simulink model "parnas_pacemaker_v7"  (R2017b)
settings: Solver=FixedStepAuto  StartTime=0.0  StopTime=10  FixedStep=1E-3  RelTol=1e-3  EnableMultiTasking=on
undefined symbols (not defined in the file): A0, A1, D0, D1, D10, D11, D12, D13, D2, D3, D4, D5, D6, D7, D8, D9, magnitude, PTA0, PTA1, PTA2, PTB2, PTB23, PTB3, PTB9, PTC16, PTC17, PTC2, PTC3, PTC4, PTD0, PTD1, PTD2, PTD3
libraries: frdmk64flib x19, etargetslib x2
settings Model: ExtModeTrigDuration=5  Creator=fahadbandali  LastModifiedBy=fahadbandali
settings OptimizationCC: PassReuseOutputArgsAs=Individual arguments  MaxStackSize=64
settings DebuggingCC: ParameterTunabilityLossMsg=error
settings HardwareCC: ProdBitPerPointer=32  ProdBitPerSizeT=32  ProdBitPerPtrDiffT=32  ProdLargestAtomicInteger=Long  ProdLargestAtomicFloat=Double  ProdWordSize=32  ProdHWDeviceType=ARM Compatible->ARM Cortex
settings SFSimCC: MATLABDynamicMemAlloc=off
settings RTWCC: SystemTargetFile=ert.tlc  HardwareBoard=NXP FRDM-K64F  TemplateMakefile=ert_default_tmf  GenerateReport=on  Toolchain=GNU Tools for ARM Embedded Processors  IncludeHyperlinkInReport=on  LaunchReport=on  GenerateTraceInfo=on  GenerateTraceReport=on  GenerateTraceReportSl=on  GenerateTraceReportSf=on  GenerateTraceReportEml=on
settings CodeAppCC: ForceParamTrailComments=on  IgnoreCustomStorageClasses=off  OperatorAnnotations=on  SimulinkDataObjDesc=on  SFDataObjDesc=on  InsertBlockDesc=on

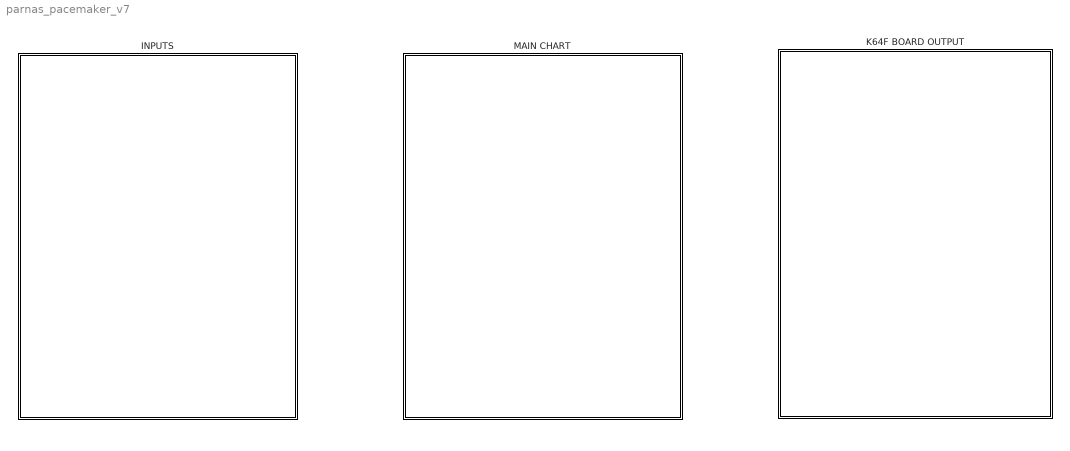
== system parnas_pacemaker_v7 ==
  "INPUTS " : Subsystem
  "K64F BOARD OUTPUT " : Subsystem
  "MAIN CHART " : Subsystem

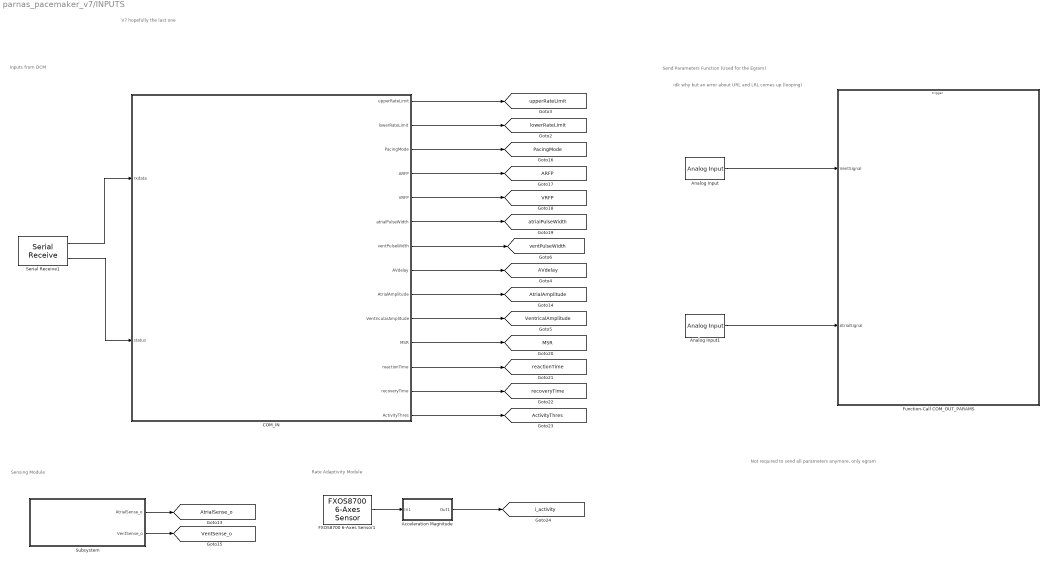
== system parnas_pacemaker_v7/INPUTS  ==
  note: Not required to send all parameters anymore, only egram
  note: V7 hopefully the last one
  note: idk why but an error about URL and LRL comes up (looping)
  note: Send Parameters Function (Used for the Egram)
  note: Inputs from DCM
  note: Rate Adaptivity Module
  note: Sensing Module
  Acceleration Magnitude : Subsystem
  Analog Input : frdmk64flib/Analog Input  Whichpin=PTB3 (A1)  SampleTime=-1
      settings: SourceProductName=Simulink Coder Support Package for NXP FRDM-K64F Board
  Analog Input1 : frdmk64flib/Analog Input  Whichpin=PTB2 (A0)  SampleTime=-1
      settings: SourceProductName=Simulink Coder Support Package for NXP FRDM-K64F Board
  COM_IN : Stateflow chart  TreatAsAtomicUnit=on
  FXOS8700 6-Axes Sensor1 : frdmk64flib/FXOS8700 6-Axes Sensor  Activesensor=Accelerometer only  ODR=800Hz  HybridODR=400Hz  Accelfullrange=-4g to +4g  SampleTime=-1
      settings: SourceProductName=Simulink Coder Support Package for NXP FRDM-K64F Board
  Function-Call COM_OUT_PARAMS : Subsystem  TreatAsAtomicUnit=on
  Serial Receive1 : frdmk64flib/Serial Receive  SCIModule=0  Baudrate=uint32(9600)  Parity=None  StopBits=1  HardwareFlowControl=None  ByteOrder=LittleEndian  DataType=uint8  DataLength=30  BlockingMode=off  OutputStatus=on  SampleTime=-1
      settings: SourceProductName=Simulink Coder Support Package for NXP FRDM-K64F Board
  Subsystem : Subsystem
  tag scope: ARFP=global, AVdelay=global, ActivityThres=global, AtrialAmplitude=global, AtrialSense_o=global, MSR=global, PacingMode=global, VRFP=global, VentSense_o=global, VentricalAmplitude=global, atrialPulseWidth=global, i_activity=global, lowerRateLimit=global, reactionTime=global, recoveryTime=global, upperRateLimit=global, ventPulseWidth=global
  wires:
  Subsystem/2("VentSense_o ") -> [VentSense_o]
  Subsystem/1("AtrialSense_o ") -> [AtrialSense_o]
  FXOS8700 6-Axes Sensor1/1 -> Acceleration Magnitude/1(In1)
  COM_IN/3(PacingMode) -> [PacingMode]
  COM_IN/4(ARFP) -> [ARFP]
  COM_IN/5(VRFP) -> [VRFP]
  COM_IN/6(atrialPulseWidth) -> [atrialPulseWidth]
  COM_IN/8(AVdelay) -> [AVdelay]
  COM_IN/9(AtrialAmplitude) -> [AtrialAmplitude]
  COM_IN/10(VentricularAmplitude) -> [VentricalAmplitude]
  COM_IN/11(MSR) -> [MSR]
  COM_IN/12(reactionTime) -> [reactionTime]
  COM_IN/13(recoveryTime) -> [recoveryTime]
  COM_IN/14(ActivityThres) -> [ActivityThres]
  Serial Receive1/1 -> COM_IN/1(rxdata)
  Serial Receive1/2 -> COM_IN/2(status)
  Analog Input1/1 -> Function-Call COM_OUT_PARAMS/2(AtrialSignal)
  Analog Input/1 -> Function-Call COM_OUT_PARAMS/1(VentSignal)
  COM_IN/1(upperRateLimit) -> [upperRateLimit]
  COM_IN/2(lowerRateLimit) -> [lowerRateLimit]
  COM_IN/7(ventPulseWidth) -> [ventPulseWidth]
  Acceleration Magnitude/1(Out1) -> [i_activity]

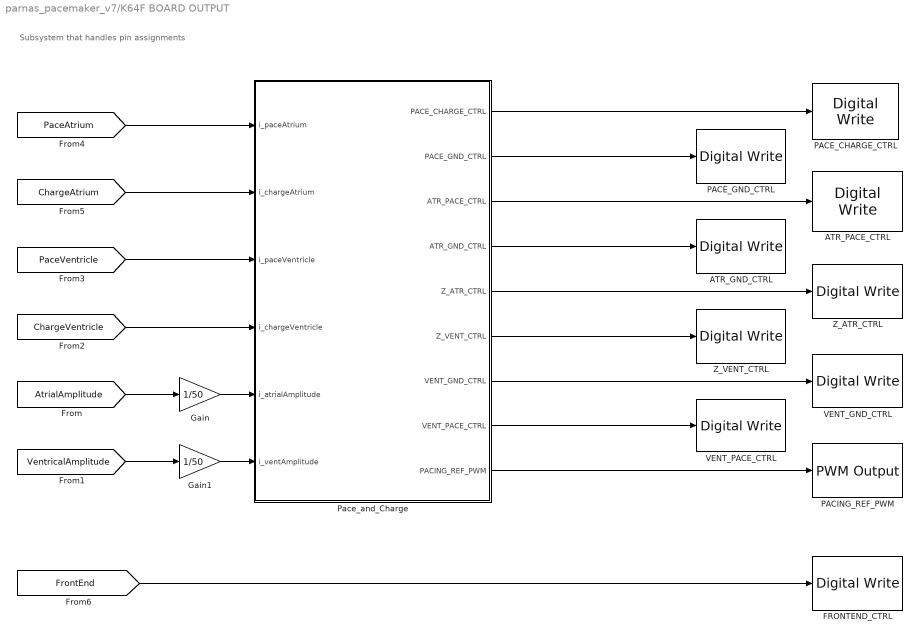
== system parnas_pacemaker_v7/K64F BOARD OUTPUT  ==
  note: Subsystem that handles pin assignments
  " ATR_GND_CTRL" : frdmk64flib/Digital Write  Whichpin=PTD2 (D11)
      settings: SourceProductName=Simulink Coder Support Package for NXP FRDM-K64F Board
  " ATR_PACE_CTRL" : frdmk64flib/Digital Write  Whichpin=PTA0 (D8)
      settings: SourceProductName=Simulink Coder Support Package for NXP FRDM-K64F Board
  " PACE_GND_CTRL" : frdmk64flib/Digital Write  Whichpin=PTD0 (D10)
      settings: SourceProductName=Simulink Coder Support Package for NXP FRDM-K64F Board
  " VENT_PACE_CTRL" : frdmk64flib/Digital Write  Whichpin=PTC4 (D9)
      settings: SourceProductName=Simulink Coder Support Package for NXP FRDM-K64F Board
  "FRONTEND_CTRL " : frdmk64flib/Digital Write  Whichpin=PTD1 (D13)
      settings: SourceProductName=Simulink Coder Support Package for NXP FRDM-K64F Board
  Gain : Gain  Gain=1/50  OutDataTypeStr=uint16
  Gain1 : Gain  Gain=1/50  OutDataTypeStr=uint16
  PACE_CHARGE_CTRL : frdmk64flib/Digital Write  Whichpin=PTB9 (D2)
      settings: SourceProductName=Simulink Coder Support Package for NXP FRDM-K64F Board
  PACING_REF_PWM : frdmk64flib/PWM Output  Whichpin=PTA2 (D5)  InitialFrequency=2000  InitialDutyCycle=0
      settings: SourceProductName=Simulink Coder Support Package for NXP FRDM-K64F Board
  Pace_and_Charge : Stateflow chart  TreatAsAtomicUnit=on
  "VENT_GND_CTRL " : frdmk64flib/Digital Write  Whichpin=PTD3 (D12)
      settings: SourceProductName=Simulink Coder Support Package for NXP FRDM-K64F Board
  Z_ATR_CTRL : frdmk64flib/Digital Write  Whichpin=PTB23 (D4)
      settings: SourceProductName=Simulink Coder Support Package for NXP FRDM-K64F Board
  Z_VENT_CTRL : frdmk64flib/Digital Write  Whichpin=PTC3 (D7)
      settings: SourceProductName=Simulink Coder Support Package for NXP FRDM-K64F Board
  wires:
  Pace_and_Charge/1(PACE_CHARGE_CTRL) -> PACE_CHARGE_CTRL/1
  Pace_and_Charge/2(PACE_GND_CTRL) -> " PACE_GND_CTRL"/1
  Pace_and_Charge/3(ATR_PACE_CTRL) -> " ATR_PACE_CTRL"/1
  [PaceAtrium] -> Pace_and_Charge/1(i_paceAtrium)
  [PaceVentricle] -> Pace_and_Charge/3(i_paceVentricle)
  Pace_and_Charge/4(ATR_GND_CTRL) -> " ATR_GND_CTRL"/1
  Pace_and_Charge/5(Z_ATR_CTRL) -> Z_ATR_CTRL/1
  Pace_and_Charge/6(Z_VENT_CTRL) -> Z_VENT_CTRL/1
  Pace_and_Charge/7(VENT_GND_CTRL) -> "VENT_GND_CTRL "/1
  Pace_and_Charge/8(VENT_PACE_CTRL) -> " VENT_PACE_CTRL"/1
  Pace_and_Charge/9(PACING_REF_PWM) -> PACING_REF_PWM/1
  [ChargeAtrium] -> Pace_and_Charge/2(i_chargeAtrium)
  [ChargeVentricle] -> Pace_and_Charge/4(i_chargeVentricle)
  [AtrialAmplitude] -> Gain/1
  Gain/1 -> Pace_and_Charge/5(i_atrialAmplitude)
  [VentricalAmplitude] -> Gain1/1
  Gain1/1 -> Pace_and_Charge/6(i_ventAmplitude)
  [FrontEnd] -> "FRONTEND_CTRL "/1

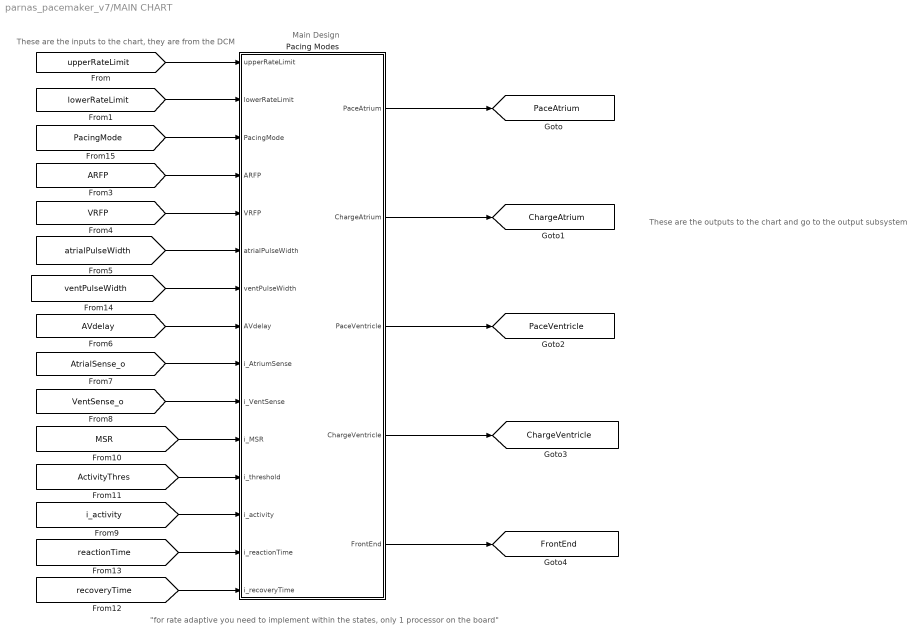
== system parnas_pacemaker_v7/MAIN CHART  ==
  note: These are the outputs to the chart and go to the output subsystem
  note: These are the inputs to the chart, they are from the DCM
  note: Main Design
  note: "for rate adaptive you need to implement within the states, only 1 processor on the board"
  Pacing Modes : Stateflow chart  TreatAsAtomicUnit=on
  tag scope: ChargeAtrium=global, ChargeVentricle=global, FrontEnd=global, PaceAtrium=global, PaceVentricle=global
  wires:
  [PacingMode] -> Pacing Modes/3(PacingMode)
  [AVdelay] -> Pacing Modes/8(AVdelay)
  [VentSense_o] -> Pacing Modes/10(i_VentSense)
  [upperRateLimit] -> Pacing Modes/1(upperRateLimit)
  Pacing Modes/3(PaceVentricle) -> [PaceVentricle]
  [atrialPulseWidth] -> Pacing Modes/6(atrialPulseWidth)
  Pacing Modes/5(FrontEnd) -> [FrontEnd]
  [AtrialSense_o] -> Pacing Modes/9(i_AtriumSense)
  [VRFP] -> Pacing Modes/5(VRFP)
  [ARFP] -> Pacing Modes/4(ARFP)
  Pacing Modes/2(ChargeAtrium) -> [ChargeAtrium]
  Pacing Modes/1(PaceAtrium) -> [PaceAtrium]
  [MSR] -> Pacing Modes/11(i_MSR)
  [ActivityThres] -> Pacing Modes/12(i_threshold)
  [lowerRateLimit] -> Pacing Modes/2(lowerRateLimit)
  [i_activity] -> Pacing Modes/13(i_activity)
  Pacing Modes/4(ChargeVentricle) -> [ChargeVentricle]
  [ventPulseWidth] -> Pacing Modes/7(ventPulseWidth)
  [recoveryTime] -> Pacing Modes/15(i_recoveryTime)
  [reactionTime] -> Pacing Modes/14(i_reactionTime)

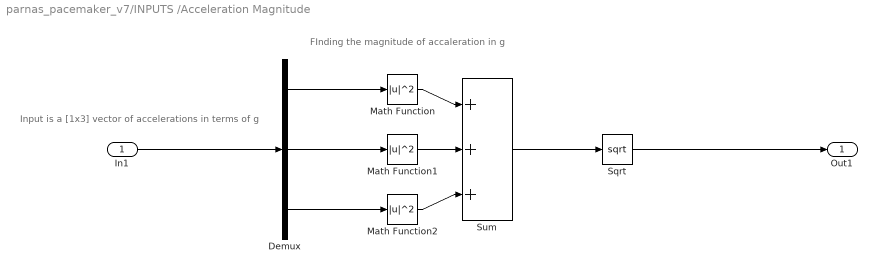
== system parnas_pacemaker_v7/INPUTS /Acceleration Magnitude ==
  note: FInding the magnitude of accaleration in g
  note: Input is a [1x3] vector of accelerations in terms of g
  In1 : Inport
  Demux : Demux  Outputs=3
  Math Function : Math  Operator=magnitude^2  OutDataTypeStr=double  SaturateOnIntegerOverflow=on
  Math Function1 : Math  Operator=magnitude^2  OutDataTypeStr=double  SaturateOnIntegerOverflow=on
  Math Function2 : Math  Operator=magnitude^2  OutDataTypeStr=double  SaturateOnIntegerOverflow=on
  Sqrt : Sqrt  OutputSignalType=real  OutDataTypeStr=uint16  SaturateOnIntegerOverflow=on
  Sum : Sum  Inputs=+|+|+  OutDataTypeStr=double
  Out1 : Outport  OutDataTypeStr=uint16
  wires:
  In1/1 -> Demux/1
  Demux/1 -> Math Function/1
  Demux/3 -> Math Function2/1
  Demux/2 -> Math Function1/1
  Math Function/1 -> Sum/1
  Math Function1/1 -> Sum/2
  Math Function2/1 -> Sum/3
  Sum/1 -> Sqrt/1
  Sqrt/1 -> Out1/1

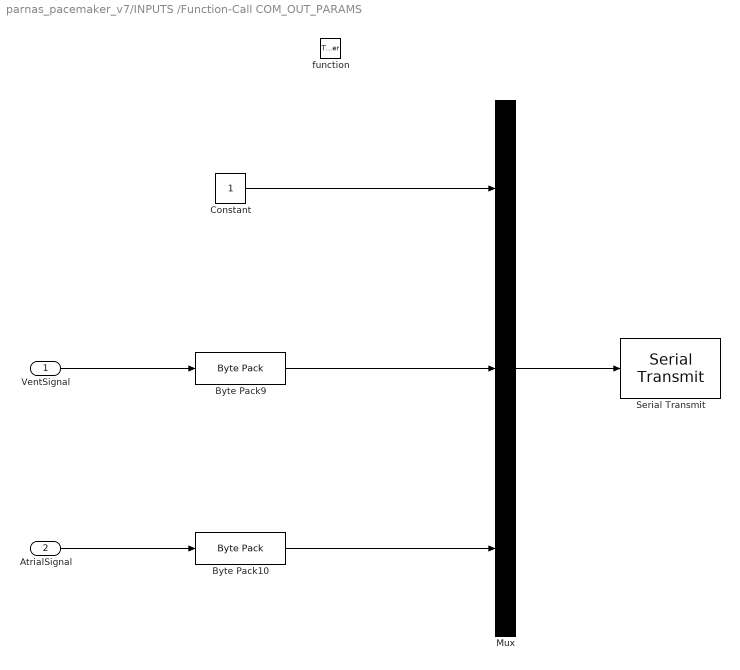
== system parnas_pacemaker_v7/INPUTS /Function-Call COM_OUT_PARAMS ==
  VentSignal : Inport
  AtrialSignal : Inport  Port=2
  function : TriggerPort  TriggerType=function-call  IsSimulinkFunction=on  FunctionName=eegram  VariantControl=Variant
  Byte Pack10 : etargetslib/Byte Pack  datatypes={'double'}  byteAlign=1
  Byte Pack9 : etargetslib/Byte Pack  datatypes={'double'}  byteAlign=1
  Constant : Constant  OutDataTypeStr=uint8
  Mux : Mux  Inputs=3
  Serial Transmit : frdmk64flib/Serial Transmit  SCIModule=0  Baudrate=uint32(9600)  Parity=None  StopBits=1  HardwareFlowControl=None  ByteOrder=LittleEndian  BlockingMode=on  OutputStatus=off
      settings: SourceProductName=Simulink Coder Support Package for NXP FRDM-K64F Board
  wires:
  Mux/1 -> Serial Transmit/1
  Byte Pack9/1 -> Mux/2
  AtrialSignal/1 -> Byte Pack10/1
  VentSignal/1 -> Byte Pack9/1
  Byte Pack10/1 -> Mux/3
  Constant/1 -> Mux/1

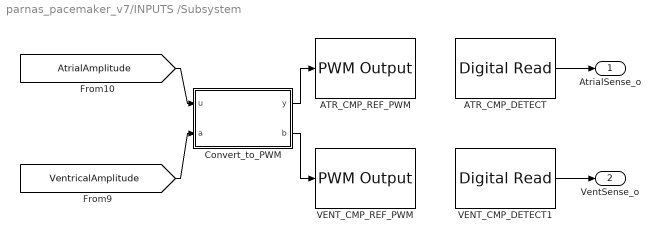
== system parnas_pacemaker_v7/INPUTS /Subsystem ==
  " ATR_CMP_DETECT" : frdmk64flib/Digital Read  Whichpin=PTC16 (D0)  SampleTime=-1
      settings: SourceProductName=Simulink Coder Support Package for NXP FRDM-K64F Board
  " VENT_CMP_DETECT1" : frdmk64flib/Digital Read  Whichpin=PTC17 (D1)  SampleTime=-1
      settings: SourceProductName=Simulink Coder Support Package for NXP FRDM-K64F Board
  ATR_CMP_REF_PWM : frdmk64flib/PWM Output  Whichpin=PTC2 (D6)  InitialFrequency=2000  InitialDutyCycle=0
      settings: SourceProductName=Simulink Coder Support Package for NXP FRDM-K64F Board
  Convert_to_PWM : MATLAB Function  TreatAsAtomicUnit=on
  VENT_CMP_REF_PWM : frdmk64flib/PWM Output  Whichpin=PTA1 (D3)  InitialFrequency=2000  InitialDutyCycle=0
      settings: SourceProductName=Simulink Coder Support Package for NXP FRDM-K64F Board
  "AtrialSense_o " : Outport  OutDataTypeStr=boolean
  "VentSense_o " : Outport  Port=2  OutDataTypeStr=boolean
  wires:
  " ATR_CMP_DETECT"/1 -> "AtrialSense_o "/1
  [VentricalAmplitude] -> Convert_to_PWM/2(a)
  Convert_to_PWM/1(y) -> ATR_CMP_REF_PWM/1
  " VENT_CMP_DETECT1"/1 -> "VentSense_o "/1
  [AtrialAmplitude] -> Convert_to_PWM/1(u)
  Convert_to_PWM/2(b) -> VENT_CMP_REF_PWM/1

== stateflow chart parnas_pacemaker_v7/INPUTS /COM_IN ==
  settings: executeAtInitialization=1
  state SET_PARAM
    entry:
    %setting the values of the parameters
    %using serial communication
    upperRateLimit = typecast(rxdata(3:4), 'uint16');
    lowerRateLimit = typecast(rxdata(5:6), 'uint16');
    PacingMode = typecast(rxdata(7:8), 'uint16');
    ARFP = typecast(rxdata(9:10), 'uint16');
    VRFP = typecast(rxdata(11:12), 'uint16');
    atrialPulseWidth = typecast(rxdata(13:14), 'uint16');
    ventPulseWidth = typecast(rxdata(15:16), 'uint16');
    AVdelay = typecast(rxdata(17:18), 'uint16');
    AtrialAmplitude = typecast(rxdata(19:20), 'uint16');
    VentricularAmplitude = typecast(rxdata(21:22), 'uint16');
    MSR = typecast(rxdata(23:24), 'uint16');
    reactionTime = typecast(rxdata(25:26), 'uint16');
    recoveryTime = typecast(rxdata(27:28), 'uint16');
    ActivityThres = typecast(rxdata(29:30), 'uint16');
    %need to add more parameters
  state INITIAL
    entry:
    %initialize the starting value of the model
    upperRateLimit = 0;
    lowerRateLimit = 0;
    PacingMode = 0;
    ARFP = 0;
    VRFP = 0;
    atrialPulseWidth = 0;
    ventPulseWidth = 0;
    AVdelay = 0;
    AtrialAmplitude = 0;
    VentricularAmplitude = 0;
    MSR = 0;
    reactionTime = 0;
    recoveryTime = 0;
    ActivityThres = 0;
  state STANDBY
    entry:
    %waiting for COM
  state ECHO_PARAM
    entry:
    eegram();
  SET_PARAM -> STANDBY
  (default) -> INITIAL
  (junction 16) -> STANDBY [order 2]
  (junction 17) -> SET_PARAM : [rxdata(2) == hex2dec('55')]
  INITIAL -> STANDBY
  STANDBY -> (junction 16) [order 1] : [status == 0]
  (junction 16) -> (junction 17) [order 1] : [rxdata(1) == hex2dec('16')]
  ECHO_PARAM -> (junction 16) [order 2] : [status == 0]
  ECHO_PARAM -> STANDBY [order 1] : [status == 32]
  STANDBY -> ECHO_PARAM [order 2] : [status == 32]
  data: upperRateLimit output uint16; lowerRateLimit output uint16; PacingMode output uint16; ARFP output uint16; VRFP output uint16; atrialPulseWidth output uint16; ventPulseWidth output uint16; AVdelay output uint16; AtrialAmplitude output uint16; VentricularAmplitude output uint16; rxdata input uint8 size=[30;1]; status input uint8 size=[1;1]; MSR output uint16; reactionTime output uint16; recoveryTime output uint16; ActivityThres output uint16

== stateflow chart parnas_pacemaker_v7/MAIN CHART /Pacing Modes ==
  state DOOR
    note: RATE ADAPTIVE
    state DOO_APACE
      entry:
      PaceAtrium = true;
      PaceVentricle = false;
      ChargeAtrium = false;
      ChargeVentricle = false;
    state DOO_ACHARGE
      entry:
      PaceAtrium = false;
      PaceVentricle = false;
      ChargeAtrium = true;
      ChargeVentricle = false;
      state Start
        entry:
        prevLRL = lowerRateLimitR;
      state FInd_Next_LRL
        entry:
        %finding the response factor (1-16)
        respFactor = i_activity*(4/sqrt(3));
        %finding the new required LRL
        nextLRL = (i_MSR - lowerRateLimit)*(respFactor/16) + lowerRateLimit;
      state Lower_Rate
        entry:
        rateChange = (i_MSR+prevLRL)/2  - lowerRateLimit + 1;
        lowerRateLimitR = floor(prevLRL - (rateChange*60)/(lowerRateLimit*i_recoveryTime));
      state Increase_Rate
        entry:
        rateChange = nextLRL - lowerRateLimit; %find the change in rate
        lowerRateLimitR = prevLRL + (rateChange*60)/(lowerRateLimit*i_reactionTime);
      state Maintain_Rate
        entry:
        lowerRateLimitR  = prevLRL;
      (default) -> DOOR.DOO_ACHARGE.Start
      DOOR.DOO_ACHARGE.Start -> DOOR.DOO_ACHARGE.FInd_Next_LRL [order 1] : [i_activity >= i_threshold]
      DOOR.DOO_ACHARGE.Start -> (junction 443) [order 2] : [i_activity < i_threshold]
      (junction 443) -> DOOR.DOO_ACHARGE.Lower_Rate [order 1] : [prevLRL > lowerRateLimit]
      DOOR.DOO_ACHARGE.FInd_Next_LRL -> DOOR.DOO_ACHARGE.Maintain_Rate [order 2] : [nextLRL <= prevLRL]
      (junction 443) -> DOOR.DOO_ACHARGE.Maintain_Rate [order 2] : [prevLRL <= lowerRateLimit]
      DOOR.DOO_ACHARGE.FInd_Next_LRL -> DOOR.DOO_ACHARGE.Increase_Rate [order 1] : [nextLRL > prevLRL]
    note: RATE ADAPTIVE
    note: DOOR
    note: This state is responsible for pacing both the ventricle and atrium
    state DOO_VPACE
      entry:
      PaceAtrium = false;
      PaceVentricle = true;
      ChargeAtrium = false;
      ChargeVentricle = false;
    state DOO_VCHARGE
      entry:
      PaceAtrium = false;
      PaceVentricle = false;
      ChargeAtrium = false;
      ChargeVentricle = true;
    note: the whole state should be (lowerRateLimit)
    (default) -> DOOR.DOO_ACHARGE : {lowerRateLimitR = lowerRateLimit}
    DOOR.DOO_ACHARGE -> DOOR.DOO_APACE : [after((60000/lowerRateLimitR -AVdelay-ventPulseWidth-atrialPulseWidth), msec)]
    DOOR.DOO_VPACE -> DOOR.DOO_ACHARGE : [after(ventPulseWidth,msec)]
    DOOR.DOO_APACE -> DOOR.DOO_VCHARGE : [after(atrialPulseWidth, msec)]
    DOOR.DOO_VCHARGE -> DOOR.DOO_VPACE : [after(AVdelay,msec)]
  state AAIR
    state AAI_Charge
      entry:
      PaceAtrium = false;
      PaceVentricle = false;
      ChargeVentricle = false;
      ChargeAtrium = true;
      FrontEnd = true;
      state Start
        entry:
        prevLRL = lowerRateLimitR;
      state FInd_Next_LRL
        entry:
        %finding the response factor (1-16)
        respFactor = i_activity*(4/sqrt(3));
        %finding the new required LRL
        nextLRL = (i_MSR - lowerRateLimit)*(respFactor/16) + lowerRateLimit;
      state Lower_Rate
        entry:
        rateChange = (i_MSR+prevLRL)/2  - lowerRateLimit + 1;
        lowerRateLimitR = floor(prevLRL - (rateChange*60)/(lowerRateLimit*i_recoveryTime));
      state Increase_Rate
        entry:
        rateChange = nextLRL - lowerRateLimit; %find the change in rate
        lowerRateLimitR = prevLRL + (rateChange*60)/(lowerRateLimit*i_reactionTime);
      state Maintain_Rate
        entry:
        lowerRateLimitR  = prevLRL;
      (default) -> AAIR.AAI_Charge.Start
      AAIR.AAI_Charge.Start -> AAIR.AAI_Charge.FInd_Next_LRL [order 1] : [i_activity >= i_threshold]
      AAIR.AAI_Charge.Start -> (junction 456) [order 2] : [i_activity < i_threshold]
      (junction 456) -> AAIR.AAI_Charge.Lower_Rate [order 1] : [prevLRL > lowerRateLimit]
      AAIR.AAI_Charge.FInd_Next_LRL -> AAIR.AAI_Charge.Maintain_Rate [order 2] : [nextLRL <= prevLRL]
      (junction 456) -> AAIR.AAI_Charge.Maintain_Rate [order 2] : [prevLRL <= lowerRateLimit]
      AAIR.AAI_Charge.FInd_Next_LRL -> AAIR.AAI_Charge.Increase_Rate [order 1] : [nextLRL > prevLRL]
    note: RATE ADAPTIVE
    note: AAIR
    note: This state is responsible for sensing a pulse in the atrium
        | Initially charging and if a pace is sensed, move to refractor state
        |
        | It stays here for RFP msec and goes back to the initial state,
        | this gives time for the next pulse to appear. If the pulse is not detected
        |
        | It goes to AAI_Pace where a pace is sent and goes back to the refractor state
    state Refractor_AAI
      entry:
      PaceAtrium = false;
      PaceVentricle = false;
      ChargeVentricle = false;
      ChargeAtrium = true;
      FrontEnd = false;
    state AAI_Pace
      entry:
      ChargeAtrium = false;
      ChargeVentricle = false;
      PaceVentricle = false;
      PaceAtrium = true;
      FrontEnd = false;
    (default) -> AAIR.AAI_Charge : {lowerRateLimitR = lowerRateLimit}
    AAIR.AAI_Charge -> AAIR.Refractor_AAI [order 2] : [i_AtriumSense == true]{offset = 0}
    AAIR.AAI_Charge -> AAIR.AAI_Pace [order 1] : [after(60000/lowerRateLimitR -ARFP-offset,msec)]
    AAIR.Refractor_AAI -> AAIR.AAI_Charge : [after(ARFP,msec)]
    AAIR.AAI_Pace -> AAIR.Refractor_AAI : [after(atrialPulseWidth, msec)]{offset = atrialPulseWidth}
  state VVIR
    state VVI_Charge2
      entry:
      PaceAtrium = false;
      PaceVentricle = false;
      ChargeAtrium = false;
      ChargeVentricle = true;
      FrontEnd = true;
      state Start
        entry:
        prevLRL = lowerRateLimitR;
      state FInd_Next_LRL
        entry:
        %finding the response factor (1-16)
        respFactor = i_activity*(4/sqrt(3));
        %finding the new required LRL
        nextLRL = (i_MSR - lowerRateLimit)*(respFactor/16) + lowerRateLimit;
      state Lower_Rate
        entry:
        rateChange = (i_MSR+prevLRL)/2  - lowerRateLimit + 1;
        lowerRateLimitR = floor(prevLRL - (rateChange*60)/(lowerRateLimit*i_recoveryTime));
      state Increase_Rate
        entry:
        rateChange = nextLRL - lowerRateLimit; %find the change in rate
        lowerRateLimitR = prevLRL + (rateChange*60)/(lowerRateLimit*i_reactionTime);
      state Maintain_Rate
        entry:
        lowerRateLimitR  = prevLRL;
      (default) -> VVIR.VVI_Charge2.Start
      VVIR.VVI_Charge2.Start -> VVIR.VVI_Charge2.FInd_Next_LRL [order 1] : [i_activity >= i_threshold]
      VVIR.VVI_Charge2.Start -> (junction 428) [order 2] : [i_activity < i_threshold]
      (junction 428) -> VVIR.VVI_Charge2.Lower_Rate [order 1] : [prevLRL > lowerRateLimit]
      VVIR.VVI_Charge2.FInd_Next_LRL -> VVIR.VVI_Charge2.Maintain_Rate [order 2] : [nextLRL <= prevLRL]
      (junction 428) -> VVIR.VVI_Charge2.Maintain_Rate [order 2] : [prevLRL <= lowerRateLimit]
      VVIR.VVI_Charge2.FInd_Next_LRL -> VVIR.VVI_Charge2.Increase_Rate [order 1] : [nextLRL > prevLRL]
    note: RATE ADAPTIVE
    note: VVIR
    note: This state is responsible for sensing a pulse in the ventrical
        | Initially charging and if a pace is sensed, move to refractor state
        |
        | It stays here for RFP msec and goes back to the initial state,
        | this gives time for the next pulse to appear. If the pulse is not detected
        |
        | It goes to VVI_Pace where a pace is sent and goes back to the refractor state
    state Refractor_VVI
      entry:
      PaceAtrium = false;
      PaceVentricle = false;
      ChargeVentricle = true;
      ChargeAtrium = false;
      FrontEnd = false;
    state VVI_Pace1
      entry:
      ChargeAtrium = false;
      ChargeVentricle = false;
      PaceVentricle = true;
      PaceAtrium = false;
      FrontEnd = false;
    (default) -> VVI_Charge2 : {lowerRateLimitR = lowerRateLimit}
    VVI_Charge2 -> VVI_Pace1 [order 1] : [after(60000/lowerRateLimitR-VRFP-offset,msec)]
    VVI_Charge2 -> VVIR.Refractor_VVI [order 2] : [i_VentSense == true]{offset = 0}
    VVIR.Refractor_VVI -> VVI_Charge2 : [after(VRFP,msec)]
    VVI_Pace1 -> VVIR.Refractor_VVI : [after(ventPulseWidth, msec)]{offset = ventPulseWidth}
  state AOOR
    note: AOOR
    state AOO_Pace
      entry:
      ChargeAtrium = false;
      ChargeVentricle = false;
      PaceVentricle = false;
      PaceAtrium = true;
    state AOO_Charge
      entry:
      PaceAtrium = false;
      PaceVentricle = false;
      ChargeVentricle = false;
      ChargeAtrium = true;
      state Start
        entry:
        prevLRL = lowerRateLimitR;
      state FInd_Next_LRL
        entry:
        %finding the response factor (1-16)
        respFactor = i_activity*(4/sqrt(3));
        %finding the new required LRL
        nextLRL = (i_MSR - lowerRateLimit)*(respFactor/16) + lowerRateLimit;
      state Lower_Rate
        entry:
        rateChange = (i_MSR+prevLRL)/2  - lowerRateLimit + 1;
        lowerRateLimitR = floor(prevLRL - (rateChange*60)/(lowerRateLimit*i_recoveryTime));
      state Increase_Rate
        entry:
        rateChange = nextLRL - lowerRateLimit; %find the change in rate
        lowerRateLimitR = prevLRL + (rateChange*60)/(lowerRateLimit*i_reactionTime);
      state Maintain_Rate
        entry:
        lowerRateLimitR  = prevLRL;
      (default) -> AOOR.AOO_Charge.Start
      AOOR.AOO_Charge.Start -> AOOR.AOO_Charge.FInd_Next_LRL [order 1] : [i_activity >= i_threshold]
      AOOR.AOO_Charge.Start -> (junction 469) [order 2] : [i_activity < i_threshold]
      (junction 469) -> AOOR.AOO_Charge.Lower_Rate [order 1] : [prevLRL > lowerRateLimit]
      AOOR.AOO_Charge.FInd_Next_LRL -> AOOR.AOO_Charge.Maintain_Rate [order 2] : [nextLRL <= prevLRL]
      (junction 469) -> AOOR.AOO_Charge.Maintain_Rate [order 2] : [prevLRL <= lowerRateLimit]
      AOOR.AOO_Charge.FInd_Next_LRL -> AOOR.AOO_Charge.Increase_Rate [order 1] : [nextLRL > prevLRL]
    note: Paces the Atrium for one cycle
        | the cycle is lowerRateLimit
        |
        | So it charges for lowerRate-pulsewidth
        | and it paces for pulseWidth amount of time
    note: RATE ADAPTIVE
    AOOR.AOO_Charge -> AOOR.AOO_Pace : [after((60000/lowerRateLimitR-atrialPulseWidth), msec)]
    (default) -> AOOR.AOO_Charge : {lowerRateLimitR = lowerRateLimit}
    AOOR.AOO_Pace -> AOOR.AOO_Charge : [after(atrialPulseWidth, msec)]
  state VOOR
    note: RATE ADAPTIVE
    state VOO_Pace
      entry:
      ChargeAtrium = false;
      ChargeVentricle = false;
      PaceAtrium = false;
      PaceVentricle = true;
    note: VOOR
    state VOO_Charge
      entry:
      PaceAtrium = false;
      PaceVentricle = false;
      ChargeAtrium = false;
      ChargeVentricle = true;
      state Start
        entry:
        prevLRL = lowerRateLimitR;
      state FInd_Next_LRL
        entry:
        %finding the response factor (1-16)
        respFactor = i_activity*(4/sqrt(3));
        %finding the new required LRL
        nextLRL = (i_MSR - lowerRateLimit)*(respFactor/16) + lowerRateLimit;
      state Lower_Rate
        entry:
        rateChange = (i_MSR+prevLRL)/2  - lowerRateLimit + 1;
        lowerRateLimitR = floor(prevLRL - (rateChange*60)/(lowerRateLimit*i_recoveryTime));
      state Increase_Rate
        entry:
        rateChange = nextLRL - lowerRateLimit; %find the change in rate
        lowerRateLimitR = prevLRL + (rateChange*60)/(lowerRateLimit*i_reactionTime);
      state Maintain_Rate
        entry:
        lowerRateLimitR  = prevLRL;
      (default) -> VOOR.VOO_Charge.Start
      VOOR.VOO_Charge.Start -> VOOR.VOO_Charge.FInd_Next_LRL [order 1] : [i_activity >= i_threshold]
      VOOR.VOO_Charge.Start -> (junction 394) [order 2] : [i_activity < i_threshold]
      (junction 394) -> VOOR.VOO_Charge.Lower_Rate [order 1] : [prevLRL > lowerRateLimit]
      VOOR.VOO_Charge.FInd_Next_LRL -> VOOR.VOO_Charge.Maintain_Rate [order 2] : [nextLRL <= prevLRL]
      (junction 394) -> VOOR.VOO_Charge.Maintain_Rate [order 2] : [prevLRL <= lowerRateLimit]
      VOOR.VOO_Charge.FInd_Next_LRL -> VOOR.VOO_Charge.Increase_Rate [order 1] : [nextLRL > prevLRL]
    note: Paces the Ventricle for one cycle
        | the cycle is lowerRateLimit
        |
        | So it charges for lowerRate-pulsewidth
        | and it paces for pulseWidth amount of time
    note: RATE ADAPTIVE
    VOOR.VOO_Charge -> VOOR.VOO_Pace : [after((60000/lowerRateLimitR-ventPulseWidth), msec)]
    (default) -> VOOR.VOO_Charge : {lowerRateLimitR = lowerRateLimit}
    VOOR.VOO_Pace -> VOOR.VOO_Charge : [after(ventPulseWidth, msec)]
  state Rest
    entry:
    offset = 0;
  state AOO
    note: AOO
    state AOO_Pace
      entry:
      ChargeAtrium = false;
      ChargeVentricle = false;
      PaceVentricle = false;
      PaceAtrium = true;
    state AOO_Charge
      entry:
      PaceAtrium = false;
      PaceVentricle = false;
      ChargeVentricle = false;
      ChargeAtrium = true;
    note: Paces the Atrium for one cycle
        | the cycle is lowerRateLimit
        |
        | So it charges for lowerRate-pulsewidth
        | and it paces for pulseWidth amount of time
    AOO.AOO_Charge -> AOO.AOO_Pace : [after((60000/lowerRateLimit-atrialPulseWidth), msec)]
    (default) -> AOO.AOO_Pace
    AOO.AOO_Pace -> AOO.AOO_Charge : [after(atrialPulseWidth, msec)]
  state VOO
    state VOO_Pace
      entry:
      ChargeAtrium = false;
      ChargeVentricle = false;
      PaceAtrium = false;
      PaceVentricle = true;
    note: VOO
    state VOO_Charge
      entry:
      PaceAtrium = false;
      PaceVentricle = false;
      ChargeAtrium = false;
      ChargeVentricle = true;
    note: Paces the Ventricle for one cycle
        | the cycle is lowerRateLimit
        |
        | So it charges for lowerRate-pulsewidth
        | and it paces for pulseWidth amount of time
    VOO.VOO_Charge -> VOO.VOO_Pace : [after((60000/lowerRateLimit-ventPulseWidth), msec)]
    (default) -> VOO.VOO_Charge
    VOO.VOO_Pace -> VOO.VOO_Charge : [after(ventPulseWidth, msec)]
  state VVI
    state VVI_Charge
      entry:
      PaceAtrium = false;
      PaceVentricle = false;
      ChargeAtrium = false;
      ChargeVentricle = true;
      FrontEnd = true;
    note: VVI
    note: This state is responsible for sensing a pulse in the ventrical
        | Initially charging and if a pace is sensed, move to refractor state
        |
        | It stays here for RFP msec and goes back to the initial state,
        | this gives time for the next pulse to appear. If the pulse is not detected
        |
        | It goes to VVI_Pace where a pace is sent and goes back to the refractor state
    state VVI_Pace
      entry:
      ChargeAtrium = false;
      ChargeVentricle = false;
      PaceAtrium = false;
      PaceVentricle = true;
      FrontEnd = true;
    state Refractor_VVI
      entry:
      PaceAtrium = false;
      PaceVentricle = false;
      ChargeAtrium = false;
      ChargeVentricle = true;
      FrontEnd = true;
    (default) -> VVI_Charge
    VVI_Charge -> VVI.Refractor_VVI [order 2] : [i_VentSense == true]{offset = 0}
    VVI_Charge -> VVI_Pace [order 1] : [after((60000/lowerRateLimit-VRFP-offset),msec)]
    VVI.Refractor_VVI -> VVI_Charge : [after(VRFP,msec)]
    VVI_Pace -> VVI.Refractor_VVI : [after(ventPulseWidth,msec)]{offset = ventPulseWidth}
  state AAI
    state AAI_Charge
      entry:
      PaceAtrium = false;
      PaceVentricle = false;
      ChargeVentricle = false;
      ChargeAtrium = true;
      FrontEnd = true;
    note: AAI
    note: This state is responsible for sensing a pulse in the atrium
        | Initially charging and if a pace is sensed, move to refractor state
        |
        | It stays here for RFP msec and goes back to the initial state,
        | this gives time for the next pulse to appear. If the pulse is not detected
        |
        | It goes to AAI_Pace where a pace is sent and goes back to the refractor state
    state AAI_Pace
      entry:
      ChargeAtrium = false;
      ChargeVentricle = false;
      PaceVentricle = false;
      PaceAtrium = true;
      FrontEnd = false;
    state Refractor_AAI
      entry:
      PaceAtrium = false;
      PaceVentricle = false;
      ChargeVentricle = false;
      ChargeAtrium = true;
      FrontEnd = false;
    (default) -> AAI.AAI_Charge
    AAI.AAI_Charge -> AAI.AAI_Pace [order 1] : [after((60000/lowerRateLimit-ARFP-offset),msec)]
    AAI.AAI_Charge -> AAI.Refractor_AAI [order 2] : [i_AtriumSense == true]{offset = 0}
    AAI.Refractor_AAI -> AAI.AAI_Charge : [after(ARFP,msec)]
    AAI.AAI_Pace -> AAI.Refractor_AAI : [after(atrialPulseWidth, msec)]{offset = atrialPulseWidth}
  state DOO
    state DOO_APACE
      entry:
      PaceAtrium = true;
      PaceVentricle = false;
      ChargeAtrium = false;
      ChargeVentricle = false;
    state DOO_ACHARGE
      entry:
      PaceAtrium = false;
      PaceVentricle = false;
      ChargeAtrium = true;
      ChargeVentricle = false;
    note: DOO
    note: This state is responsible for pacing both the ventricle and atrium
    state DOO_VPACE
      entry:
      PaceAtrium = false;
      PaceVentricle = true;
      ChargeAtrium = false;
      ChargeVentricle = false;
    state DOO_VCHARGE
      entry:
      PaceAtrium = false;
      PaceVentricle = false;
      ChargeAtrium = false;
      ChargeVentricle = true;
    note: the whole state should be (lowerRateLimit)
    (default) -> DOO.DOO_ACHARGE
    DOO.DOO_ACHARGE -> DOO.DOO_APACE : [after((60000/lowerRateLimit-AVdelay-ventPulseWidth-atrialPulseWidth), msec)]
    DOO.DOO_VPACE -> DOO.DOO_ACHARGE : [after(ventPulseWidth,msec)]
    DOO.DOO_APACE -> DOO.DOO_VCHARGE : [after(atrialPulseWidth, msec)]
    DOO.DOO_VCHARGE -> DOO.DOO_VPACE : [after(AVdelay,msec)]
  Rest -> DOOR [order 1] : [PacingMode == 10]
  DOOR -> Rest : [PacingMode ~= 10]
  AAIR -> Rest : [PacingMode ~= 9]
  Rest -> AAIR [order 10] : [PacingMode == 9]
  VVIR -> Rest : [PacingMode ~= 8]
  Rest -> VVIR [order 9] : [PacingMode == 8]
  Rest -> AOOR [order 8] : [PacingMode == 7]
  Rest -> VOOR [order 7] : [PacingMode == 6]
  VOOR -> Rest : [PacingMode ~= 6]
  AOOR -> Rest : [PacingMode ~= 7]
  (default) -> Rest
  Rest -> VOO [order 2] : [PacingMode == 1]
  AOO -> Rest : [PacingMode ~= 2]
  VOO -> Rest : [PacingMode ~= 1]
  VVI -> Rest : [PacingMode ~= 3]
  Rest -> AOO [order 3] : [PacingMode == 2]
  Rest -> VVI [order 5] : [PacingMode == 3]
  DOO -> Rest : [PacingMode ~= 5]
  Rest -> DOO [order 6] : [PacingMode == 5]
  AAI -> Rest : [PacingMode ~= 4]
  Rest -> AAI [order 4] : [PacingMode == 4]
  data: PaceAtrium output boolean; upperRateLimit input uint16; lowerRateLimit input uint16; ChargeAtrium output boolean; PaceVentricle output boolean; ChargeVentricle output boolean; PacingMode input uint16; ARFP input uint16; FrontEnd output boolean; VRFP input uint16; atrialPulseWidth input uint16; ventPulseWidth input uint16; AVdelay input uint16; i_AtriumSense input boolean; i_VentSense input boolean; offset local uint16; lowerRateLimitR local uint16; prevLRL local uint16; rateChange local uint16; nextLRL local uint16; i_MSR input uint16; i_threshold input uint16; i_activity input uint16; i_reactionTime input uint16; respFactor local uint16; i_recoveryTime input uint16

== stateflow chart parnas_pacemaker_v7/K64F BOARD OUTPUT /Pace_and_Charge ==
  state Rest
    entry:
    ATR_PACE_CTRL = false;
    VENT_PACE_CTRL = false;
    PACING_REF_PWM = 0;
    PACE_CHARGE_CTRL = false;
    PACE_GND_CTRL = false;
    Z_ATR_CTRL = false;
    Z_VENT_CTRL = false;
    ATR_GND_CTRL = false;
    VENT_GND_CTRL = false;
  state Charge_Atr_Paced_Atr
    %Charge C22 for atrial pulse
    %Just recieved atrial pulse
    entry:
    ATR_PACE_CTRL = false;
    VENT_PACE_CTRL = false;
    PACING_REF_PWM = i_atrialAmplitude;
    PACE_CHARGE_CTRL = true;
    %Discharging Blocking Capacitor
    PACE_GND_CTRL = true;
    Z_ATR_CTRL = false;
    Z_VENT_CTRL = false;
    ATR_GND_CTRL = true;
    VENT_GND_CTRL = false;
  state Charge_Vent_Paced_Vent
    %Charge C22 for vent pulse
    %Just recieved vent pulse
    entry:
    ATR_PACE_CTRL = false;
    VENT_PACE_CTRL = false;
    PACING_REF_PWM = i_ventAmplitude;
    PACE_CHARGE_CTRL = true;
    %Dishcharging Blocking Capacitor
    PACE_GND_CTRL = true;
    Z_ATR_CTRL = false;
    Z_VENT_CTRL = false;
    ATR_GND_CTRL = false;
    VENT_GND_CTRL = true;
  state Atrial_Pace
    entry:
    %seting pins for an atrial pace
    PACE_CHARGE_CTRL = false;
    PACE_GND_CTRL = true;
    ATR_PACE_CTRL = true;
    ATR_GND_CTRL = false;
    Z_ATR_CTRL = false;
    Z_VENT_CTRL = false;
    VENT_GND_CTRL = false;
    VENT_PACE_CTRL = false;
  state Ventricle_Pace
    entry:
    %setting pins for a ventricle pace
    PACE_CHARGE_CTRL = false;
    PACE_GND_CTRL = true;
    ATR_PACE_CTRL = false;
    ATR_GND_CTRL = false;
    Z_ATR_CTRL = false;
    Z_VENT_CTRL = false;
    VENT_GND_CTRL = false;
    VENT_PACE_CTRL = true;
  state Charge_Vent_Paced_Atr
    entry:
    %Charge C22 for ventricular pulse
    %Just recieved atrial pulse
    ATR_PACE_CTRL = false;
    VENT_PACE_CTRL = false;
    PACING_REF_PWM = i_ventAmplitude;
    PACE_CHARGE_CTRL = true;
    %Set up C21 for paced atrium
    PACE_GND_CTRL = true;
    Z_ATR_CTRL = false;
    Z_VENT_CTRL = false;
    ATR_GND_CTRL = true;
    VENT_GND_CTRL = false;
  state Charge_Atr_Paced_Vent
    entry:
    %Charge C22 for atrial pulse
    %Just recieved ventricular pulse
    ATR_PACE_CTRL = false;
    VENT_PACE_CTRL = false;
    PACING_REF_PWM = i_atrialAmplitude;
    PACE_CHARGE_CTRL = true;
    %Set up C21 for paced ventricle
    PACE_GND_CTRL = true;
    Z_ATR_CTRL = false;
    Z_VENT_CTRL = false;
    ATR_GND_CTRL = false;
    VENT_GND_CTRL = true;
  (default) -> Rest
  Rest -> Charge_Vent_Paced_Vent [order 1] : [i_chargeVentricle == true]
  Rest -> Charge_Atr_Paced_Atr [order 2] : [i_chargeAtrium == true]
  Charge_Atr_Paced_Vent -> Rest [order 2] : [i_chargeAtrium == false]
  Charge_Vent_Paced_Atr -> Rest [order 2] : [i_chargeVentricle == false]
  Charge_Atr_Paced_Atr -> Rest [order 2] : [i_chargeAtrium == false]
  Charge_Vent_Paced_Vent -> Rest [order 2] : [i_chargeVentricle == false]
  Ventricle_Pace -> Charge_Vent_Paced_Vent [order 1] : [(i_paceVentricle == false) && (i_chargeVentricle ==true)]
  Charge_Vent_Paced_Vent -> Ventricle_Pace [order 1] : [i_paceVentricle == true]
  Charge_Atr_Paced_Atr -> Atrial_Pace [order 1] : [i_paceAtrium == true]
  Atrial_Pace -> Charge_Atr_Paced_Atr [order 1] : [(i_paceAtrium == false) && (i_chargeAtrium == true)]
  Charge_Atr_Paced_Vent -> Atrial_Pace [order 1] : [i_paceAtrium == true]
  Charge_Vent_Paced_Atr -> Ventricle_Pace [order 1] : [i_paceVentricle == true]
  Ventricle_Pace -> Charge_Atr_Paced_Vent [order 2] : [(i_paceVentricle == false) && (i_chargeAtrium == true)]
  Atrial_Pace -> Charge_Vent_Paced_Atr [order 2] : [(i_paceAtrium == false) && (i_chargeVentricle == true)]
  data: i_paceAtrium input boolean; i_chargeAtrium input boolean; i_paceVentricle input boolean; PACE_CHARGE_CTRL output boolean; PACE_GND_CTRL output boolean; ATR_PACE_CTRL output boolean; ATR_GND_CTRL output boolean; Z_ATR_CTRL output boolean; Z_VENT_CTRL output boolean; VENT_GND_CTRL output boolean; VENT_PACE_CTRL output boolean; PACING_REF_PWM output uint16; i_chargeVentricle input boolean; i_atrialAmplitude input uint16; i_ventAmplitude input uint16

== matlab function parnas_pacemaker_v7/INPUTS /Subsystem/Convert_to_PWM ==
  data: u input; y output; a input; b output
function [y,b] = fcn(u, a)

y = floor(u/50);
b = floor(a/50);
